simulink model "Motor_CD"  (R2020a)
settings: Solver=VariableStepAuto  StartTime=0.0  StopTime=5  RelTol=1e-3
values from neighbouring files (symbols this model uses):
  A = [0, 1 ... (first row only)    [Nomoto.m]
  B = [0 ... (first row only)    [Nomoto.m]
  K = 0.185    [Nomoto.m]
undefined symbols (not defined in the file or in its folder): F, p
libraries: simulink x1
settings Model: Creator=luis  LastModifiedBy=micro microndas

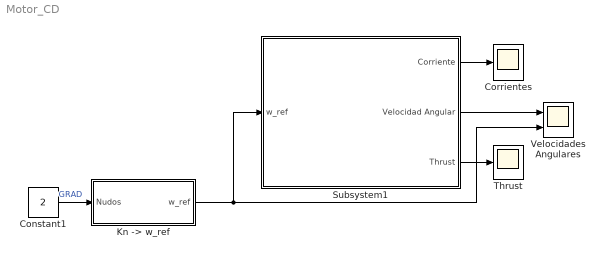
== system Motor_CD ==
  Constant1 : Constant  Value=2
  "Corrientes " : Scope
  "Kn -> w_ref" : Subsystem
  Subsystem1 : Subsystem
  Thrust : Scope
  "Velocidades Angulares " : Scope  NumInputPorts=2
  wires:
  Subsystem1/1(Corriente) -> "Corrientes "/1
  Subsystem1/2(Velocidad Angular) -> "Velocidades Angulares "/1
  Subsystem1/3(Thrust) -> Thrust/1
  "Kn -> w_ref"/1(w_ref) -> "Velocidades Angulares "/2, Subsystem1/1(w_ref)
  Constant1/1 -> "Kn -> w_ref"/1(Nudos)  "GRAD"

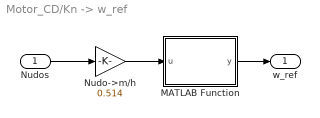
== system Motor_CD/Kn -> w_ref ==
  Nudos : Inport
  MATLAB Function : MATLAB Function  TreatAsAtomicUnit=on
  Nudo->m/h : Gain  Gain=0.514
  w_ref : Outport
  wires:
  Nudos/1 -> Nudo->m/h/1
  Nudo->m/h/1 -> MATLAB Function/1(u)
  MATLAB Function/1(y) -> w_ref/1

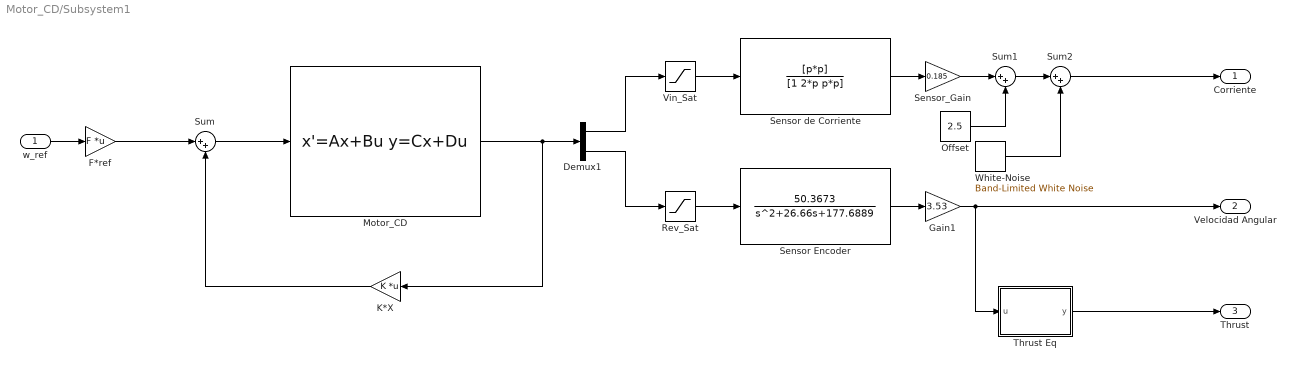
== system Motor_CD/Subsystem1 ==
  w_ref : Inport
  Demux1 : Demux  Outputs=2
  F*ref : Gain  Gain=F  Multiplication=Matrix(K*u)
  Gain1 : Gain  Gain=3.53
  K*X : Gain  Gain=K  Multiplication=Matrix(K*u)
  Motor_CD : StateSpace  A=A  B=B  C=eye(2)  D=[0;0]  InitialCondition=0  ContinuousStateAttributes={'i_t', 'w_t'}
  Offset : Constant  Value=2.5
  Rev_Sat : Saturate  UpperLimit=7500  LowerLimit=0
  Sensor Encoder : TransferFcn  Numerator=[50.3673]  Denominator=[1 26.66 177.6889]  ContinuousStateAttributes='Position'
  "Sensor de Corriente " : TransferFcn  Numerator=[p*p]  Denominator=[1 2*p p*p]  ContinuousStateAttributes='Corriente'
  Sensor_Gain : Gain  Gain=0.185
  Sum : Sum  Inputs=|++
  Sum1 : Sum  Inputs=|++
  Sum2 : Sum  Inputs=|++
  Thrust Eq : MATLAB Function  TreatAsAtomicUnit=on
  Vin_Sat : Saturate  UpperLimit=5  LowerLimit=-5
  White-Noise : simulink/Sources/Band-Limited White Noise  Cov=[1e-8]  Ts=0.001  seed=[23341]
  Corriente : Outport
  Velocidad Angular : Outport  Port=2
  Thrust : Outport  Port=3
  wires:
  Rev_Sat/1 -> Sensor Encoder/1
  "Sensor de Corriente "/1 -> Sensor_Gain/1
  Demux1/2 -> Rev_Sat/1
  Gain1/1 -> Velocidad Angular/1, Thrust Eq/1(u)
  Sum1/1 -> Sum2/1
  K*X/1 -> Sum/2
  Demux1/1 -> Vin_Sat/1
  Motor_CD/1 -> K*X/1, Demux1/1
  White-Noise/1 -> Sum2/2
  Thrust Eq/1(y) -> Thrust/1
  Sum/1 -> Motor_CD/1
  Offset/1 -> Sum1/2
  F*ref/1 -> Sum/1
  Sum2/1 -> Corriente/1
  Sensor_Gain/1 -> Sum1/1
  Sensor Encoder/1 -> Gain1/1
  Vin_Sat/1 -> "Sensor de Corriente "/1
  w_ref/1 -> F*ref/1

== matlab function Motor_CD/Kn -> w_ref/MATLAB Function ==
  data: u input; y output
function y = fcn(u)
Diam = 2.0; %mts
y = u/Diam;

== matlab function Motor_CD/Subsystem1/Thrust Eq ==
  data: u input; y output
function y = Thrust_Eq(u)

% Valores para propela
    % Thrust = Thrust_Coef*( density*Rev*Rev*Diam*Diam*Diam*Diam )

    Thrust_Coef = 0.014;
    density = 1e3; %kg/mts*mts*mts
    Diam = 2.0; %mts
    
y = ( Thrust_Coef )*( density )*( u^2 )*( Diam^4 ) ;
